simulink model "MICROBOT_1_backup"  (R2015a)
settings: Solver=ode45  StartTime=0.0  StopTime=inf  FixedStep=0.001  RelTol=1e-3
values from neighbouring files (symbols this model uses):
  s = serial('COM4','BaudRate',9600,'DataBits', 8,'Terminator',13)    [start.m]
undefined symbols (not defined in the file or in its folder): board, MICROBOT_1, RootGround, RootPart, W01_2, W02_1, W03_1, W04, W05, W06, W07, W08
libraries: mblibv1 x39
settings Model: Creator=anhkh  LastModifiedBy=anhkh
settings SimMechanicsCC: VisOnUpdateDiagram=on  VisDuringSimulation=on

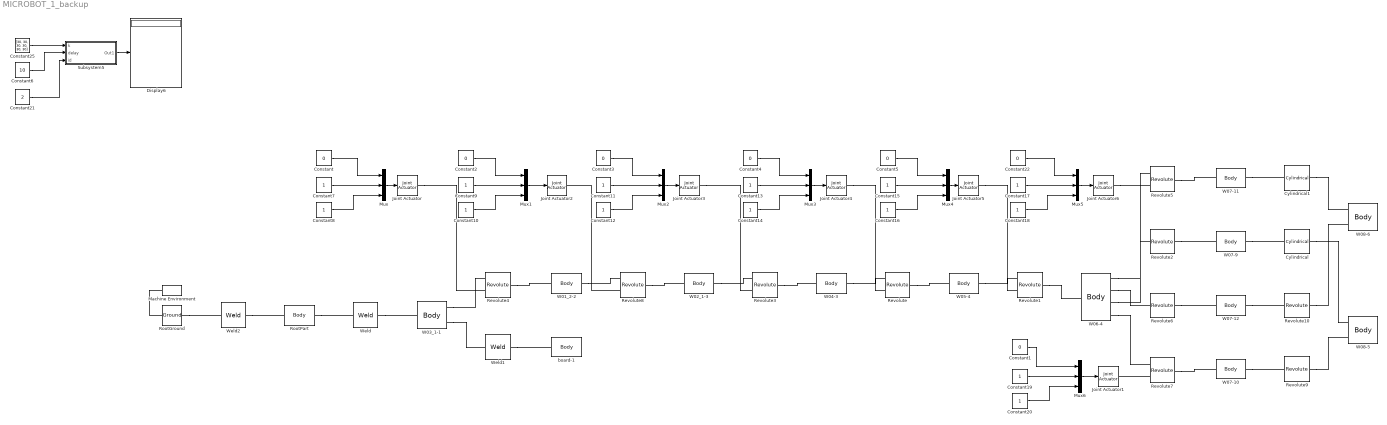
== system MICROBOT_1_backup ==
  Constant{,1..5,22} (7 alike) : Constant  Value=0
  Constant{7..20} (14 alike) : Constant
  Constant21 : Constant  Value=2
  Constant25 : Constant  Value=[30, 30, 30, 30, 30, 30]
  Constant6 : Constant  Value=10
  Cylindrical : mblibv1/Joints/Cylindrical  LConnTagsString=__newl0  RConnTagsString=__newr0  UpdateFromCAD=on  PMImportedID=W07-9:-:W08-5  NumSAPorts=0  CutJoint=off  MarkAsCut=off  Primitives=prismatic  PrimitiveProps=P1$WORLD$[0.0885398,3.2164e-12,0.996073]$prismatic#R1$WORLD$[0.0885398,3.21611e-12,0.996073]$revolute  DialogClass=JointBlock  P1Axis=[0.0885398,3.2164e-12,0.996073]  R1Axis=[0.0885398,3.21611e-12,0.996073]
  Cylindrical1 : mblibv1/Joints/Cylindrical  LConnTagsString=__newl0  RConnTagsString=__newr0  UpdateFromCAD=on  PMImportedID=W07-11:-:W08-6  NumSAPorts=0  CutJoint=off  MarkAsCut=off  Primitives=prismatic  PrimitiveProps=P1$WORLD$[-0.0885398,-3.21743e-12,-0.996073]$prismatic#R1$WORLD$[0.0885398,3.21752e-12,0.996073]$revolute  DialogClass=JointBlock  P1Axis=[-0.0885398,-3.21743e-12,-0.996073]  R1Axis=[0.0885398,3.21752e-12,0.996073]
  Display6 : Display
  Joint Actuator{,1..6} (7 alike) : mblibv1/Sensors &  Actuators/Joint Actuator  UpdateFromCAD=off  PhysicalDomain=Mechanical  PortType=blob  ActuationStyle=Motion  AngleUnits=deg  ArcVelocityUnits=deg/s  ArcAccelerationUnits=deg/s^2  CoordPositionUnits=m  VelocityUnits=m/s  AccelerationUnits=m/s^2  ForceUnits=N  TorqueUnits=N*m  ActiveIO=on  Width=3  DialogClass=MechanicalActuatorBlock  Primitive=R1  ReferenceFrame=Absolute (World)
  Machine Environment : mblibv1/Bodies/Machine Environment  PortType=env  PhysicalDomain=Mechanical  DialogTemplateClass=MECH.MachineEnvironment  SyncWhenCopied=off  Gravity=[0 -9.81 0]  GravityUnits=m/s^2  GravityAsSignal=off  Dimensionality=Auto-detect  AnalysisType=Forward dynamics  LinearAssemblyTolerance=1e-3  LinearAssemblyToleranceUnits=m  AngularAssemblyTolerance=1e-3  AngularAssemblyToleranceUnits=rad  ConstraintSolverType=Stabilizing  ConstraintRelTolerance=1e-4  ConstraintAbsTolerance=1e-4  UseRobustSingularityHandling=off  RedundancyAnalysisToleranceType=Automatically select tolerance  RedundancyAnalysisTolerance=1e-14  StatePerturbationType=Fixed  PerturbationSize=1e-5  VisualizeMachine=on  BodyVisualizationType=Use model default body geometries  BodyColorSelMode=Use model default  DefaultBodyColor=[1 0 0]
  Mux{,1..6} (7 alike) : Mux  Inputs=3
  Revolute : mblibv1/Joints/Revolute  LConnTagsString=__newl0|SA1  RConnTagsString=__newr0  UpdateFromCAD=on  PMImportedID=W04-3:-:W05-4  NumSAPorts=1  CutJoint=off  MarkAsCut=off  Primitives=prismatic  PrimitiveProps=R1$WORLD$[1.97265e-12,1,0]$revolute  DialogClass=JointBlock  R1Axis=[1.97265e-12,1,0]
  Revolute1 : mblibv1/Joints/Revolute  LConnTagsString=__newl0|SA1  RConnTagsString=__newr0  UpdateFromCAD=on  PMImportedID=W05-4:-:W06-4  NumSAPorts=1  CutJoint=off  MarkAsCut=off  Primitives=prismatic  PrimitiveProps=R1$WORLD$[0.996073,-1.96452e-12,-0.0885398]$revolute  DialogClass=JointBlock  R1Axis=[0.996073,-1.96452e-12,-0.0885398]
  Revolute10 : mblibv1/Joints/Revolute  LConnTagsString=__newl0  RConnTagsString=__newr0  UpdateFromCAD=on  PMImportedID=W07-12:-:W08-6  NumSAPorts=0  CutJoint=off  MarkAsCut=off  Primitives=prismatic  PrimitiveProps=R1$WORLD$[0.0885398,3.21754e-12,0.996073]$revolute  DialogClass=JointBlock  R1Axis=[0.0885398,3.21754e-12,0.996073]
  Revolute2 : mblibv1/Joints/Revolute  LConnTagsString=__newl0  RConnTagsString=__newr0  UpdateFromCAD=on  PMImportedID=W06-4:-:W07-9  NumSAPorts=0  CutJoint=off  MarkAsCut=off  Primitives=prismatic  PrimitiveProps=R1$WORLD$[-0.0885398,-3.21743e-12,-0.996073]$revolute  DialogClass=JointBlock  R1Axis=[-0.0885398,-3.21743e-12,-0.996073]
  Revolute3 : mblibv1/Joints/Revolute  LConnTagsString=__newl0|SA1  RConnTagsString=__newr0  UpdateFromCAD=on  PMImportedID=W02_1-3:-:W04-3  NumSAPorts=1  CutJoint=off  MarkAsCut=off  Primitives=prismatic  PrimitiveProps=R1$WORLD$[1.97263e-12,1,0]$revolute  DialogClass=JointBlock  R1Axis=[1.97263e-12,1,0]
  Revolute4 : mblibv1/Joints/Revolute  LConnTagsString=__newl0|SA1  RConnTagsString=__newr0  UpdateFromCAD=on  PMImportedID=W01_2-2:-:W03_1-1  NumSAPorts=1  CutJoint=off  MarkAsCut=off  Primitives=prismatic  PrimitiveProps=R1$WORLD$[0,0,-1]$revolute  DialogClass=JointBlock  R1Axis=[0,0,-1]
  Revolute5 : mblibv1/Joints/Revolute  LConnTagsString=__newl0|SA1  RConnTagsString=__newr0  UpdateFromCAD=on  PMImportedID=W06-4:-:W07-11  NumSAPorts=1  CutJoint=off  MarkAsCut=off  Primitives=prismatic  PrimitiveProps=R1$WORLD$[-0.0885398,-3.21743e-12,-0.996073]$revolute  DialogClass=JointBlock  R1Axis=[-0.0885398,-3.21743e-12,-0.996073]
  Revolute6 : mblibv1/Joints/Revolute  LConnTagsString=__newl0  RConnTagsString=__newr0  UpdateFromCAD=on  PMImportedID=W06-4:-:W07-12  NumSAPorts=0  CutJoint=off  MarkAsCut=off  Primitives=prismatic  PrimitiveProps=R1$WORLD$[-0.0885398,-3.21743e-12,-0.996073]$revolute  DialogClass=JointBlock  R1Axis=[-0.0885398,-3.21743e-12,-0.996073]
  Revolute7 : mblibv1/Joints/Revolute  LConnTagsString=__newl0|SA1  RConnTagsString=__newr0  UpdateFromCAD=on  PMImportedID=W06-4:-:W07-10  NumSAPorts=1  CutJoint=off  MarkAsCut=off  Primitives=prismatic  PrimitiveProps=R1$WORLD$[-0.0885398,-3.21743e-12,-0.996073]$revolute  DialogClass=JointBlock  R1Axis=[-0.0885398,-3.21743e-12,-0.996073]
  Revolute8 : mblibv1/Joints/Revolute  LConnTagsString=__newl0|SA1  RConnTagsString=__newr0  UpdateFromCAD=on  PMImportedID=W01_2-2:-:W02_1-3  NumSAPorts=1  CutJoint=off  MarkAsCut=off  Primitives=prismatic  PrimitiveProps=R1$WORLD$[-1.9721e-12,-1,0]$revolute  DialogClass=JointBlock  R1Axis=[-1.9721e-12,-1,0]
  Revolute9 : mblibv1/Joints/Revolute  LConnTagsString=__newl0  RConnTagsString=__newr0  UpdateFromCAD=on  PMImportedID=W07-10:-:W08-5  NumSAPorts=0  CutJoint=off  MarkAsCut=off  Primitives=prismatic  PrimitiveProps=R1$WORLD$[0.0885398,3.2164e-12,0.996073]$revolute  DialogClass=JointBlock  R1Axis=[0.0885398,3.2164e-12,0.996073]
  RootGround : mblibv1/Bodies/Ground  UpdateFromCAD=on  PMImportedID=RootGround  LeftPortType=env  RightPortType=workingframe  PhysicalDomain=Mechanical  DialogClass=GroundBlock  CoordPosition=[-0.110803,0.40847,0.0544949]  CoordPositionUnits=m  StateVectorMgrId=3  MachineId=[4 0]  ShowEnvPort=on  ParameterChecksum=[2064798137, 1484770623, 251117345, 3844192694]  TopologyChecksum=[3823588316, 2441359055, 4135265906, 3916664184]
  RootPart : mblibv1/Bodies/Body  LConnTagsString=CS3  RConnTagsString=CS2  UpdateFromCAD=on  PMImportedID=MICROBOT_1/RootPart  DialogClass=MechanicalBodyBlock  Mass=0  MassUnits=kg  InertiaUnits=kg*m^2  Inertia=[0,0,0;0,0,0;0,0,0]  Shape=Cylinder  ShapeDims=[1 1]  ShapeUnits=m  ShapeUse=false  Density=1  DensityUnits=kg/m^3  DensityUse=false  GraphicsMode=MACHINE_DEFAULT  BodyColorSelMode=MACHINE_DEFAULT  BodyColor=[1;0;0]  AttachedToCS=CS1  CG=Right$CG$[-0.110803 0.40847 0.0544949]$WORLD$WORLD$m$[1 0 0;0 1 0;0 0 1]$3x3 Transform$rad$WORLD$false$MICROBOT_1/RootPart::CG(AUTOGEN)  WorkingFrames=Right$CS1$[0 0 0]$WORLD$WORLD$m$[1 0 0;0 1 0;0 0 1]$3x3 Transform$rad$WORLD$false$MICROBOT_1/RootPart::CS1(AUTOGEN)#Right$CS2$[-0.107087 0.143871 0.0371879]$WORLD$WORLD$m$[1 0 0;0 1 0;0 0 1]$3x3 Transform$rad$WORLD$true$MICROBOT_1/RootPart:-:W03_1-1::MICROBOT_1/RootPart(AUTOGEN)#Left$CS3$[-0.110803 0.40847 0.0544949]$WORLD$WORLD$m$[1 0 0;0 1 0;0 0 1]$3x3 Transform$rad$WORLD$true$MICROBOT_1/RootPart:-:RootGround::MICROBOT_1/RootPart(AUTOGEN)  CGPos=[-0.110803 0.40847 0.0544949]  CGRot=[1 0 0;0 1 0;0 0 1]  CS0Pos=[]  CS0Rot=[]  CS1Pos=[0 0 0]  CS1Rot=[1 0 0;0 1 0;0 0 1]  CS2Pos=[-0.107087 0.143871 0.0371879]  CS2Rot=[1 0 0;0 1 0;0 0 1]  CS3Pos=[-0.110803 0.40847 0.0544949]  CS3Rot=[1 0 0;0 1 0;0 0 1]  CS4Pos=[]  CS4Rot=[]  CS5Pos=[]  CS5Rot=[]  CS6Pos=[]  CS6Rot=[]  CS7Pos=[]  CS7Rot=[]  CS8Pos=[]  CS8Rot=[]  CS9Pos=[]  CS9Rot=[]  CS10Pos=[]  CS10Rot=[]  CS11Pos=[]  CS11Rot=[]  CS12Pos=[]  CS12Rot=[]  CS13Pos=[]  CS13Rot=[]  CS14Pos=[]  CS14Rot=[]  CS15Pos=[]  CS15Rot=[]  CS16Pos=[]  CS16Rot=[]  CS17Pos=[]  CS17Rot=[]  CS18Pos=[]  CS18Rot=[]  CS19Pos=[]  CS19Rot=[]  CS20Pos=[]  CS20Rot=[]
  Subsystem5 : Subsystem
  W01_2-2 : mblibv1/Bodies/Body  LConnTagsString=CS3  RConnTagsString=CS2  UpdateFromCAD=on  PMImportedID=W01_2-2  DialogClass=MechanicalBodyBlock  Mass=3.41752  MassUnits=kg  InertiaUnits=kg*m^2  Inertia=[0.0156091,-9.74217e-10,-8.96339e-09;-9.74217e-10,0.0136555,0.00112438;-8.96339e-09,0.00112438,0.0159365]  Shape=Cylinder  ShapeDims=[1 1]  ShapeUnits=m  ShapeUse=false  Density=1  DensityUnits=kg/m^3  DensityUse=false  GraphicsMode=GFXFILE  GraphicsFileName=MICROBOT_1 - W01_2-2.STL  BodyColorSelMode=COLORPALETTE  BodyColor=[0.792157;0.819608;0.933333]  AttachedToCS=CS1  CG=Right$CG$[-0.15354 0.221184 0.150881]$WORLD$WORLD$m$[1.9721e-12 1 0;1 -1.9721e-12 0;0 0 -1]$3x3 Transform$rad$WORLD$false$W01_2-2::CG(AUTOGEN)  WorkingFrames=Right$CS1$[-0.157087 0.221184 0.193]$WORLD$WORLD$m$[1.9721e-12 1 0;1 -1.9721e-12 0;0 0 -1]$3x3 Transform$rad$WORLD$false$W01_2-2::CS1(AUTOGEN)#Right$CS2$[-0.107087 0.252684 0.243]$WORLD$WORLD$m$[1 0 0;0 1 0;0 0 1]$3x3 Transform$rad$WORLD$true$W01_2-2:-:W02_1-3::W01_2-2(AUTOGEN)#Left$CS3$[-0.107087 0.221184 0.103]$WORLD$WORLD$m$[1 0 0;0 1 0;0 0 1]$3x3 Transform$rad$WORLD$true$W01_2-2:-:W03_1-1::W01_2-2(AUTOGEN)  CGPos=[-0.15354 0.221184 0.150881]  CGRot=[1.9721e-12 1 0;1 -1.9721e-12 0;0 0 -1]  CS0Pos=[]  CS0Rot=[]  CS1Pos=[-0.157087 0.221184 0.193]  CS1Rot=[1.9721e-12 1 0;1 -1.9721e-12 0;0 0 -1]  CS2Pos=[-0.107087 0.252684 0.243]  CS2Rot=[1 0 0;0 1 0;0 0 1]  CS3Pos=[-0.107087 0.221184 0.103]  CS3Rot=[1 0 0;0 1 0;0 0 1]  CS4Pos=[]  CS4Rot=[]  CS5Pos=[]  CS5Rot=[]  CS6Pos=[]  CS6Rot=[]  CS7Pos=[]  CS7Rot=[]  CS8Pos=[]  CS8Rot=[]  CS9Pos=[]  CS9Rot=[]  CS10Pos=[]  CS10Rot=[]  CS11Pos=[]  CS11Rot=[]  CS12Pos=[]  CS12Rot=[]  CS13Pos=[]  CS13Rot=[]  CS14Pos=[]  CS14Rot=[]  CS15Pos=[]  CS15Rot=[]  CS16Pos=[]  CS16Rot=[]  CS17Pos=[]  CS17Rot=[]  CS18Pos=[]  CS18Rot=[]  CS19Pos=[]  CS19Rot=[]  CS20Pos=[]  CS20Rot=[]
  W02_1-3 : mblibv1/Bodies/Body  LConnTagsString=CS2  RConnTagsString=CS3  UpdateFromCAD=on  PMImportedID=W02_1-3  DialogClass=MechanicalBodyBlock  Mass=0.137184  MassUnits=kg  InertiaUnits=kg*m^2  Inertia=[0.000250835,-0.000173843,-1.3272e-07;-0.000173843,0.000692155,9.67815e-08;-1.3272e-07,9.67815e-08,0.000724516]  Shape=Cylinder  ShapeDims=[1 1]  ShapeUnits=m  ShapeUse=false  Density=1  DensityUnits=kg/m^3  DensityUse=false  GraphicsMode=GFXFILE  GraphicsFileName=MICROBOT_1 - W02_1-3.STL  BodyColorSelMode=COLORPALETTE  BodyColor=[0.792157;0.819608;0.933333]  AttachedToCS=CS1  CG=Right$CG$[-0.0248881 0.22102 0.249502]$WORLD$WORLD$m$[0.948668 0.316273 -1.97263e-12;-1.86984e-12 0 -1;-0.316273 0.948668 0]$3x3 Transform$rad$WORLD$false$W02_1-3::CG(AUTOGEN)  WorkingFrames=Right$CS1$[-0.0240745 0.252684 0.238257]$WORLD$WORLD$m$[0.948668 0.316273 -1.97263e-12;-1.86984e-12 0 -1;-0.316273 0.948668 0]$3x3 Transform$rad$WORLD$false$W02_1-3::CS1(AUTOGEN)#Left$CS2$[-0.107087 0.252684 0.243]$WORLD$WORLD$m$[1 0 0;0 1 0;0 0 1]$3x3 Transform$rad$WORLD$true$W01_2-2:-:W02_1-3::W02_1-3(AUTOGEN)#Right$CS3$[0.0779125 0.236184 0.243]$WORLD$WORLD$m$[1 0 0;0 1 0;0 0 1]$3x3 Transform$rad$WORLD$true$W02_1-3:-:W04-3::W02_1-3(AUTOGEN)  CGPos=[-0.0248881 0.22102 0.249502]  CGRot=[0.948668 0.316273 -1.97263e-12;-1.86984e-12 0 -1;-0.316273 0.948668 0]  CS0Pos=[]  CS0Rot=[]  CS1Pos=[-0.0240745 0.252684 0.238257]  CS1Rot=[0.948668 0.316273 -1.97263e-12;-1.86984e-12 0 -1;-0.316273 0.948668 0]  CS2Pos=[-0.107087 0.252684 0.243]  CS2Rot=[1 0 0;0 1 0;0 0 1]  CS3Pos=[0.0779125 0.236184 0.243]  CS3Rot=[1 0 0;0 1 0;0 0 1]  CS4Pos=[]  CS4Rot=[]  CS5Pos=[]  CS5Rot=[]  CS6Pos=[]  CS6Rot=[]  CS7Pos=[]  CS7Rot=[]  CS8Pos=[]  CS8Rot=[]  CS9Pos=[]  CS9Rot=[]  CS10Pos=[]  CS10Rot=[]  CS11Pos=[]  CS11Rot=[]  CS12Pos=[]  CS12Rot=[]  CS13Pos=[]  CS13Rot=[]  CS14Pos=[]  CS14Rot=[]  CS15Pos=[]  CS15Rot=[]  CS16Pos=[]  CS16Rot=[]  CS17Pos=[]  CS17Rot=[]  CS18Pos=[]  CS18Rot=[]  CS19Pos=[]  CS19Rot=[]  CS20Pos=[]  CS20Rot=[]
  W03_1-1 : mblibv1/Bodies/Body  LConnTagsString=CS2  RConnTagsString=CS3|CS4  UpdateFromCAD=on  PMImportedID=W03_1-1  DialogClass=MechanicalBodyBlock  Mass=3.89994  MassUnits=kg  InertiaUnits=kg*m^2  Inertia=[0.0172249,0,0;0,0.0322437,-3.95609e-05;0,-3.95609e-05,0.0192496]  Shape=Cylinder  ShapeDims=[1 1]  ShapeUnits=m  ShapeUse=false  Density=1  DensityUnits=kg/m^3  DensityUse=false  GraphicsMode=GFXFILE  GraphicsFileName=MICROBOT_1 - W03_1-1.STL  BodyColorSelMode=COLORPALETTE  BodyColor=[0.792157;0.819608;0.933333]  AttachedToCS=CS1  CG=Right$CG$[-0.107087 0.143871 0.0371879]$WORLD$WORLD$m$[-1 0 0;0 0 1;0 1 0]$3x3 Transform$rad$WORLD$false$W03_1-1::CG(AUTOGEN)  WorkingFrames=Right$CS1$[-0.107087 0.036184 0.04]$WORLD$WORLD$m$[-1 0 0;0 0 1;0 1 0]$3x3 Transform$rad$WORLD$false$W03_1-1::CS1(AUTOGEN)#Left$CS2$[-0.107087 0.143871 0.0371879]$WORLD$WORLD$m$[1 0 0;0 1 0;0 0 1]$3x3 Transform$rad$WORLD$true$MICROBOT_1/RootPart:-:W03_1-1::W03_1-1(AUTOGEN)#Right$CS3$[-0.107087 0.221184 0.103]$WORLD$WORLD$m$[1 0 0;0 1 0;0 0 1]$3x3 Transform$rad$WORLD$true$W01_2-2:-:W03_1-1::W03_1-1(AUTOGEN)#Right$CS4$[-0.107087 0.036184 -0.02]$WORLD$WORLD$m$[1 0 0;0 1 0;0 0 1]$3x3 Transform$rad$WORLD$true$W03_1-1:-:board-1::W03_1-1(AUTOGEN)  CGPos=[-0.107087 0.143871 0.0371879]  CGRot=[-1 0 0;0 0 1;0 1 0]  CS0Pos=[]  CS0Rot=[]  CS1Pos=[-0.107087 0.036184 0.04]  CS1Rot=[-1 0 0;0 0 1;0 1 0]  CS2Pos=[-0.107087 0.143871 0.0371879]  CS2Rot=[1 0 0;0 1 0;0 0 1]  CS3Pos=[-0.107087 0.221184 0.103]  CS3Rot=[1 0 0;0 1 0;0 0 1]  CS4Pos=[-0.107087 0.036184 -0.02]  CS4Rot=[1 0 0;0 1 0;0 0 1]  CS5Pos=[]  CS5Rot=[]  CS6Pos=[]  CS6Rot=[]  CS7Pos=[]  CS7Rot=[]  CS8Pos=[]  CS8Rot=[]  CS9Pos=[]  CS9Rot=[]  CS10Pos=[]  CS10Rot=[]  CS11Pos=[]  CS11Rot=[]  CS12Pos=[]  CS12Rot=[]  CS13Pos=[]  CS13Rot=[]  CS14Pos=[]  CS14Rot=[]  CS15Pos=[]  CS15Rot=[]  CS16Pos=[]  CS16Rot=[]  CS17Pos=[]  CS17Rot=[]  CS18Pos=[]  CS18Rot=[]  CS19Pos=[]  CS19Rot=[]  CS20Pos=[]  CS20Rot=[]
  W04-3 : mblibv1/Bodies/Body  LConnTagsString=CS2  RConnTagsString=CS3  UpdateFromCAD=on  PMImportedID=W04-3  DialogClass=MechanicalBodyBlock  Mass=0.028469  MassUnits=kg  InertiaUnits=kg*m^2  Inertia=[0.00010055,-1.1564e-07,2.98034e-07;-1.1564e-07,0.000108696,-6.97188e-07;2.98034e-07,-6.97188e-07,2.10954e-05]  Shape=Cylinder  ShapeDims=[1 1]  ShapeUnits=m  ShapeUse=false  Density=1  DensityUnits=kg/m^3  DensityUse=false  GraphicsMode=GFXFILE  GraphicsFileName=MICROBOT_1 - W04-3.STL  BodyColorSelMode=COLORPALETTE  BodyColor=[0.792157;0.819608;0.933333]  AttachedToCS=CS1  CG=Right$CG$[0.00168848 0.221868 0.236562]$WORLD$WORLD$m$[1.97265e-12 0 1;1 0 -1.97265e-12;0 1 0]$3x3 Transform$rad$WORLD$false$W04-3::CG(AUTOGEN)  WorkingFrames=Right$CS1$[0.0779125 0.221184 0.243]$WORLD$WORLD$m$[1.97265e-12 0 1;1 0 -1.97265e-12;0 1 0]$3x3 Transform$rad$WORLD$false$W04-3::CS1(AUTOGEN)#Left$CS2$[0.0779125 0.236184 0.243]$WORLD$WORLD$m$[1 0 0;0 1 0;0 0 1]$3x3 Transform$rad$WORLD$true$W02_1-3:-:W04-3::W04-3(AUTOGEN)#Right$CS3$[-0.102087 0.247184 0.243]$WORLD$WORLD$m$[1 0 0;0 1 0;0 0 1]$3x3 Transform$rad$WORLD$true$W04-3:-:W05-4::W04-3(AUTOGEN)  CGPos=[0.00168848 0.221868 0.236562]  CGRot=[1.97265e-12 0 1;1 0 -1.97265e-12;0 1 0]  CS0Pos=[]  CS0Rot=[]  CS1Pos=[0.0779125 0.221184 0.243]  CS1Rot=[1.97265e-12 0 1;1 0 -1.97265e-12;0 1 0]  CS2Pos=[0.0779125 0.236184 0.243]  CS2Rot=[1 0 0;0 1 0;0 0 1]  CS3Pos=[-0.102087 0.247184 0.243]  CS3Rot=[1 0 0;0 1 0;0 0 1]  CS4Pos=[]  CS4Rot=[]  CS5Pos=[]  CS5Rot=[]  CS6Pos=[]  CS6Rot=[]  CS7Pos=[]  CS7Rot=[]  CS8Pos=[]  CS8Rot=[]  CS9Pos=[]  CS9Rot=[]  CS10Pos=[]  CS10Rot=[]  CS11Pos=[]  CS11Rot=[]  CS12Pos=[]  CS12Rot=[]  CS13Pos=[]  CS13Rot=[]  CS14Pos=[]  CS14Rot=[]  CS15Pos=[]  CS15Rot=[]  CS16Pos=[]  CS16Rot=[]  CS17Pos=[]  CS17Rot=[]  CS18Pos=[]  CS18Rot=[]  CS19Pos=[]  CS19Rot=[]  CS20Pos=[]  CS20Rot=[]
  W05-4 : mblibv1/Bodies/Body  LConnTagsString=CS2  RConnTagsString=CS3  UpdateFromCAD=on  PMImportedID=W05-4  DialogClass=MechanicalBodyBlock  Mass=0.0114047  MassUnits=kg  InertiaUnits=kg*m^2  Inertia=[7.08852e-07,0,6.72492e-12;0,1.28223e-06,-2.77128e-11;6.72492e-12,-2.77128e-11,1.23052e-06]  Shape=Cylinder  ShapeDims=[1 1]  ShapeUnits=m  ShapeUse=false  Density=1  DensityUnits=kg/m^3  DensityUse=false  GraphicsMode=GFXFILE  GraphicsFileName=MICROBOT_1 - W05-4.STL  BodyColorSelMode=COLORPALETTE  BodyColor=[0.792157;0.819608;0.933333]  AttachedToCS=CS1  CG=Right$CG$[-0.102528 0.221184 0.243039]$WORLD$WORLD$m$[1.97271e-12 -0.996073 0.0885398;1 1.96452e-12 0;0 0.0885398 0.996073]$3x3 Transform$rad$WORLD$false$W05-4::CG(AUTOGEN)  WorkingFrames=Right$CS1$[-0.102087 0.221184 0.243]$WORLD$WORLD$m$[1.97271e-12 -0.996073 0.0885398;1 1.96452e-12 0;0 0.0885398 0.996073]$3x3 Transform$rad$WORLD$false$W05-4::CS1(AUTOGEN)#Left$CS2$[-0.102087 0.247184 0.243]$WORLD$WORLD$m$[1 0 0;0 1 0;0 0 1]$3x3 Transform$rad$WORLD$true$W04-3:-:W05-4::W05-4(AUTOGEN)#Right$CS3$[-0.103979 0.221184 0.243168]$WORLD$WORLD$m$[1 0 0;0 1 0;0 0 1]$3x3 Transform$rad$WORLD$true$W05-4:-:W06-4::W05-4(AUTOGEN)  CGPos=[-0.102528 0.221184 0.243039]  CGRot=[1.97271e-12 -0.996073 0.0885398;1 1.96452e-12 0;0 0.0885398 0.996073]  CS0Pos=[]  CS0Rot=[]  CS1Pos=[-0.102087 0.221184 0.243]  CS1Rot=[1.97271e-12 -0.996073 0.0885398;1 1.96452e-12 0;0 0.0885398 0.996073]  CS2Pos=[-0.102087 0.247184 0.243]  CS2Rot=[1 0 0;0 1 0;0 0 1]  CS3Pos=[-0.103979 0.221184 0.243168]  CS3Rot=[1 0 0;0 1 0;0 0 1]  CS4Pos=[]  CS4Rot=[]  CS5Pos=[]  CS5Rot=[]  CS6Pos=[]  CS6Rot=[]  CS7Pos=[]  CS7Rot=[]  CS8Pos=[]  CS8Rot=[]  CS9Pos=[]  CS9Rot=[]  CS10Pos=[]  CS10Rot=[]  CS11Pos=[]  CS11Rot=[]  CS12Pos=[]  CS12Rot=[]  CS13Pos=[]  CS13Rot=[]  CS14Pos=[]  CS14Rot=[]  CS15Pos=[]  CS15Rot=[]  CS16Pos=[]  CS16Rot=[]  CS17Pos=[]  CS17Rot=[]  CS18Pos=[]  CS18Rot=[]  CS19Pos=[]  CS19Rot=[]  CS20Pos=[]  CS20Rot=[]
  W06-4 : mblibv1/Bodies/Body  LConnTagsString=CS3  RConnTagsString=CS2|CS4|CS5|CS6  UpdateFromCAD=on  PMImportedID=W06-4  DialogClass=MechanicalBodyBlock  Mass=0.00360366  MassUnits=kg  InertiaUnits=kg*m^2  Inertia=[3.16611e-07,4.38162e-09,0;4.38162e-09,1.36274e-06,0;0,0,1.31379e-06]  Shape=Cylinder  ShapeDims=[1 1]  ShapeUnits=m  ShapeUse=false  Density=1  DensityUnits=kg/m^3  DensityUse=false  GraphicsMode=GFXFILE  GraphicsFileName=MICROBOT_1 - W06-4.STL  BodyColorSelMode=COLORPALETTE  BodyColor=[0.792157;0.819608;0.933333]  AttachedToCS=CS1  CG=Right$CG$[-0.0815589 0.221054 0.241175]$WORLD$WORLD$m$[-1.34635e-12 -0.996073 -0.0885398;-1 1.63765e-12 -3.21743e-12;3.34979e-12 0.0885398 -0.996073]$3x3 Transform$rad$WORLD$false$W06-4::CG(AUTOGEN)  WorkingFrames=Right$CS1$[-0.0770144 0.221184 0.240771]$WORLD$WORLD$m$[-1.34635e-12 -0.996073 -0.0885398;-1 1.63765e-12 -3.21743e-12;3.34979e-12 0.0885398 -0.996073]$3x3 Transform$rad$WORLD$false$W06-4::CS1(AUTOGEN)#Right$CS2$[-0.0797149 0.199184 0.23298]$WORLD$WORLD$m$[1 0 0;0 1 0;0 0 1]$3x3 Transform$rad$WORLD$true$W06-4:-:W07-11::W06-4(AUTOGEN)#Left$CS3$[-0.103979 0.221184 0.243168]$WORLD$WORLD$m$[1 0 0;0 1 0;0 0 1]$3x3 Transform$rad$WORLD$true$W05-4:-:W06-4::W06-4(AUTOGEN)#Right$CS4$[-0.0797149 0.191184 0.23298]$WORLD$WORLD$m$[1 0 0;0 1 0;0 0 1]$3x3 Transform$rad$WORLD$true$W06-4:-:W07-12::W06-4(AUTOGEN)#Right$CS5$[-0.0797149 0.251184 0.23298]$WORLD$WORLD$m$[1 0 0;0 1 0;0 0 1]$3x3 Transform$rad$WORLD$true$W06-4:-:W07-9::W06-4(AUTOGEN)#Right$CS6$[-0.0797149 0.243184 0.23298]$WORLD$WORLD$m$[1 0 0;0 1 0;0 0 1]$3x3 Transform$rad$WORLD$true$W06-4:-:W07-10::W06-4(AUTOGEN)  CGPos=[-0.0815589 0.221054 0.241175]  CGRot=[-1.34635e-12 -0.996073 -0.0885398;-1 1.63765e-12 -3.21743e-12;3.34979e-12 0.0885398 -0.996073]  CS0Pos=[]  CS0Rot=[]  CS1Pos=[-0.0770144 0.221184 0.240771]  CS1Rot=[-1.34635e-12 -0.996073 -0.0885398;-1 1.63765e-12 -3.21743e-12;3.34979e-12 0.0885398 -0.996073]  CS2Pos=[-0.0797149 0.199184 0.23298]  CS2Rot=[1 0 0;0 1 0;0 0 1]  CS3Pos=[-0.103979 0.221184 0.243168]  CS3Rot=[1 0 0;0 1 0;0 0 1]  CS4Pos=[-0.0797149 0.191184 0.23298]  CS4Rot=[1 0 0;0 1 0;0 0 1]  CS5Pos=[-0.0797149 0.251184 0.23298]  CS5Rot=[1 0 0;0 1 0;0 0 1]  CS6Pos=[-0.0797149 0.243184 0.23298]  CS6Rot=[1 0 0;0 1 0;0 0 1]  CS7Pos=[]  CS7Rot=[]  CS8Pos=[]  CS8Rot=[]  CS9Pos=[]  CS9Rot=[]  CS10Pos=[]  CS10Rot=[]  CS11Pos=[]  CS11Rot=[]  CS12Pos=[]  CS12Rot=[]  CS13Pos=[]  CS13Rot=[]  CS14Pos=[]  CS14Rot=[]  CS15Pos=[]  CS15Rot=[]  CS16Pos=[]  CS16Rot=[]  CS17Pos=[]  CS17Rot=[]  CS18Pos=[]  CS18Rot=[]  CS19Pos=[]  CS19Rot=[]  CS20Pos=[]  CS20Rot=[]
  W07-10 : mblibv1/Bodies/Body  LConnTagsString=CS2  RConnTagsString=CS3  UpdateFromCAD=on  PMImportedID=W07-10  DialogClass=MechanicalBodyBlock  Mass=0.00554345  MassUnits=kg  InertiaUnits=kg*m^2  Inertia=[1.25755e-06,0,0;0,1.41119e-07,0;0,0,1.16215e-06]  Shape=Cylinder  ShapeDims=[1 1]  ShapeUnits=m  ShapeUse=false  Density=1  DensityUnits=kg/m^3  DensityUse=false  GraphicsMode=GFXFILE  GraphicsFileName=MICROBOT_1 - W07-10.STL  BodyColorSelMode=COLORPALETTE  BodyColor=[0.792157;0.819608;0.933333]  AttachedToCS=CS1  CG=Right$CG$[-0.0592413 0.233684 0.239191]$WORLD$WORLD$m$[-0.430122 -0.898418 -0.0885398;-0.901961 0.431818 -3.2164e-12;0.0382331 0.0798594 -0.996073]$3x3 Transform$rad$WORLD$false$W07-10::CG(AUTOGEN)  WorkingFrames=Right$CS1$[-0.0587101 0.233684 0.245168]$WORLD$WORLD$m$[-0.430122 -0.898418 -0.0885398;-0.901961 0.431818 -3.2164e-12;0.0382331 0.0798594 -0.996073]$3x3 Transform$rad$WORLD$false$W07-10::CS1(AUTOGEN)#Left$CS2$[-0.0797149 0.243184 0.23298]$WORLD$WORLD$m$[1 0 0;0 1 0;0 0 1]$3x3 Transform$rad$WORLD$true$W06-4:-:W07-10::W07-10(AUTOGEN)#Right$CS3$[-0.0401844 0.224184 0.229466]$WORLD$WORLD$m$[1 0 0;0 1 0;0 0 1]$3x3 Transform$rad$WORLD$true$W07-10:-:W08-5::W07-10(AUTOGEN)  CGPos=[-0.0592413 0.233684 0.239191]  CGRot=[-0.430122 -0.898418 -0.0885398;-0.901961 0.431818 -3.2164e-12;0.0382331 0.0798594 -0.996073]  CS0Pos=[]  CS0Rot=[]  CS1Pos=[-0.0587101 0.233684 0.245168]  CS1Rot=[-0.430122 -0.898418 -0.0885398;-0.901961 0.431818 -3.2164e-12;0.0382331 0.0798594 -0.996073]  CS2Pos=[-0.0797149 0.243184 0.23298]  CS2Rot=[1 0 0;0 1 0;0 0 1]  CS3Pos=[-0.0401844 0.224184 0.229466]  CS3Rot=[1 0 0;0 1 0;0 0 1]  CS4Pos=[]  CS4Rot=[]  CS5Pos=[]  CS5Rot=[]  CS6Pos=[]  CS6Rot=[]  CS7Pos=[]  CS7Rot=[]  CS8Pos=[]  CS8Rot=[]  CS9Pos=[]  CS9Rot=[]  CS10Pos=[]  CS10Rot=[]  CS11Pos=[]  CS11Rot=[]  CS12Pos=[]  CS12Rot=[]  CS13Pos=[]  CS13Rot=[]  CS14Pos=[]  CS14Rot=[]  CS15Pos=[]  CS15Rot=[]  CS16Pos=[]  CS16Rot=[]  CS17Pos=[]  CS17Rot=[]  CS18Pos=[]  CS18Rot=[]  CS19Pos=[]  CS19Rot=[]  CS20Pos=[]  CS20Rot=[]
  W07-11 : mblibv1/Bodies/Body  LConnTagsString=CS3  RConnTagsString=CS2  UpdateFromCAD=on  PMImportedID=W07-11  DialogClass=MechanicalBodyBlock  Mass=0.00554345  MassUnits=kg  InertiaUnits=kg*m^2  Inertia=[1.25755e-06,0,0;0,1.41119e-07,0;0,0,1.16215e-06]  Shape=Cylinder  ShapeDims=[1 1]  ShapeUnits=m  ShapeUse=false  Density=1  DensityUnits=kg/m^3  DensityUse=false  GraphicsMode=GFXFILE  GraphicsFileName=MICROBOT_1 - W07-11.STL  BodyColorSelMode=COLORPALETTE  BodyColor=[0.792157;0.819608;0.933333]  AttachedToCS=CS1  CG=Right$CG$[-0.0592413 0.208684 0.239191]$WORLD$WORLD$m$[0.430122 -0.898418 -0.0885398;-0.901961 -0.431818 -3.21753e-12;-0.0382331 0.0798594 -0.996073]$3x3 Transform$rad$WORLD$false$W07-11::CG(AUTOGEN)  WorkingFrames=Right$CS1$[-0.0587101 0.208684 0.245168]$WORLD$WORLD$m$[0.430122 -0.898418 -0.0885398;-0.901961 -0.431818 -3.21753e-12;-0.0382331 0.0798594 -0.996073]$3x3 Transform$rad$WORLD$false$W07-11::CS1(AUTOGEN)#Right$CS2$[-0.0401844 0.218184 0.229466]$WORLD$WORLD$m$[1 0 0;0 1 0;0 0 1]$3x3 Transform$rad$WORLD$true$W07-11:-:W08-6::W07-11(AUTOGEN)#Left$CS3$[-0.0797149 0.199184 0.23298]$WORLD$WORLD$m$[1 0 0;0 1 0;0 0 1]$3x3 Transform$rad$WORLD$true$W06-4:-:W07-11::W07-11(AUTOGEN)  CGPos=[-0.0592413 0.208684 0.239191]  CGRot=[0.430122 -0.898418 -0.0885398;-0.901961 -0.431818 -3.21753e-12;-0.0382331 0.0798594 -0.996073]  CS0Pos=[]  CS0Rot=[]  CS1Pos=[-0.0587101 0.208684 0.245168]  CS1Rot=[0.430122 -0.898418 -0.0885398;-0.901961 -0.431818 -3.21753e-12;-0.0382331 0.0798594 -0.996073]  CS2Pos=[-0.0401844 0.218184 0.229466]  CS2Rot=[1 0 0;0 1 0;0 0 1]  CS3Pos=[-0.0797149 0.199184 0.23298]  CS3Rot=[1 0 0;0 1 0;0 0 1]  CS4Pos=[]  CS4Rot=[]  CS5Pos=[]  CS5Rot=[]  CS6Pos=[]  CS6Rot=[]  CS7Pos=[]  CS7Rot=[]  CS8Pos=[]  CS8Rot=[]  CS9Pos=[]  CS9Rot=[]  CS10Pos=[]  CS10Rot=[]  CS11Pos=[]  CS11Rot=[]  CS12Pos=[]  CS12Rot=[]  CS13Pos=[]  CS13Rot=[]  CS14Pos=[]  CS14Rot=[]  CS15Pos=[]  CS15Rot=[]  CS16Pos=[]  CS16Rot=[]  CS17Pos=[]  CS17Rot=[]  CS18Pos=[]  CS18Rot=[]  CS19Pos=[]  CS19Rot=[]  CS20Pos=[]  CS20Rot=[]
  W07-12 : mblibv1/Bodies/Body  LConnTagsString=CS3  RConnTagsString=CS2  UpdateFromCAD=on  PMImportedID=W07-12  DialogClass=MechanicalBodyBlock  Mass=0.00554345  MassUnits=kg  InertiaUnits=kg*m^2  Inertia=[1.25755e-06,0,0;0,1.41119e-07,0;0,0,1.16215e-06]  Shape=Cylinder  ShapeDims=[1 1]  ShapeUnits=m  ShapeUse=false  Density=1  DensityUnits=kg/m^3  DensityUse=false  GraphicsMode=GFXFILE  GraphicsFileName=MICROBOT_1 - W07-12.STL  BodyColorSelMode=COLORPALETTE  BodyColor=[0.792157;0.819608;0.933333]  AttachedToCS=CS1  CG=Right$CG$[-0.0592413 0.200684 0.239191]$WORLD$WORLD$m$[0.430122 -0.898418 -0.0885398;-0.901961 -0.431818 -3.21755e-12;-0.0382331 0.0798594 -0.996073]$3x3 Transform$rad$WORLD$false$W07-12::CG(AUTOGEN)  WorkingFrames=Right$CS1$[-0.0587101 0.200684 0.245168]$WORLD$WORLD$m$[0.430122 -0.898418 -0.0885398;-0.901961 -0.431818 -3.21755e-12;-0.0382331 0.0798594 -0.996073]$3x3 Transform$rad$WORLD$false$W07-12::CS1(AUTOGEN)#Right$CS2$[-0.0401844 0.210184 0.229466]$WORLD$WORLD$m$[1 0 0;0 1 0;0 0 1]$3x3 Transform$rad$WORLD$true$W07-12:-:W08-6::W07-12(AUTOGEN)#Left$CS3$[-0.0797149 0.191184 0.23298]$WORLD$WORLD$m$[1 0 0;0 1 0;0 0 1]$3x3 Transform$rad$WORLD$true$W06-4:-:W07-12::W07-12(AUTOGEN)  CGPos=[-0.0592413 0.200684 0.239191]  CGRot=[0.430122 -0.898418 -0.0885398;-0.901961 -0.431818 -3.21755e-12;-0.0382331 0.0798594 -0.996073]  CS0Pos=[]  CS0Rot=[]  CS1Pos=[-0.0587101 0.200684 0.245168]  CS1Rot=[0.430122 -0.898418 -0.0885398;-0.901961 -0.431818 -3.21755e-12;-0.0382331 0.0798594 -0.996073]  CS2Pos=[-0.0401844 0.210184 0.229466]  CS2Rot=[1 0 0;0 1 0;0 0 1]  CS3Pos=[-0.0797149 0.191184 0.23298]  CS3Rot=[1 0 0;0 1 0;0 0 1]  CS4Pos=[]  CS4Rot=[]  CS5Pos=[]  CS5Rot=[]  CS6Pos=[]  CS6Rot=[]  CS7Pos=[]  CS7Rot=[]  CS8Pos=[]  CS8Rot=[]  CS9Pos=[]  CS9Rot=[]  CS10Pos=[]  CS10Rot=[]  CS11Pos=[]  CS11Rot=[]  CS12Pos=[]  CS12Rot=[]  CS13Pos=[]  CS13Rot=[]  CS14Pos=[]  CS14Rot=[]  CS15Pos=[]  CS15Rot=[]  CS16Pos=[]  CS16Rot=[]  CS17Pos=[]  CS17Rot=[]  CS18Pos=[]  CS18Rot=[]  CS19Pos=[]  CS19Rot=[]  CS20Pos=[]  CS20Rot=[]
  W07-9 : mblibv1/Bodies/Body  LConnTagsString=CS2  RConnTagsString=CS3  UpdateFromCAD=on  PMImportedID=W07-9  DialogClass=MechanicalBodyBlock  Mass=0.00554345  MassUnits=kg  InertiaUnits=kg*m^2  Inertia=[1.25755e-06,0,0;0,1.41119e-07,0;0,0,1.16215e-06]  Shape=Cylinder  ShapeDims=[1 1]  ShapeUnits=m  ShapeUse=false  Density=1  DensityUnits=kg/m^3  DensityUse=false  GraphicsMode=GFXFILE  GraphicsFileName=MICROBOT_1 - W07-9.STL  BodyColorSelMode=COLORPALETTE  BodyColor=[0.792157;0.819608;0.933333]  AttachedToCS=CS1  CG=Right$CG$[-0.0592413 0.241684 0.239191]$WORLD$WORLD$m$[-0.430122 -0.898418 -0.0885398;-0.901961 0.431818 -3.2161e-12;0.0382331 0.0798594 -0.996073]$3x3 Transform$rad$WORLD$false$W07-9::CG(AUTOGEN)  WorkingFrames=Right$CS1$[-0.0587101 0.241684 0.245168]$WORLD$WORLD$m$[-0.430122 -0.898418 -0.0885398;-0.901961 0.431818 -3.2161e-12;0.0382331 0.0798594 -0.996073]$3x3 Transform$rad$WORLD$false$W07-9::CS1(AUTOGEN)#Left$CS2$[-0.0797149 0.251184 0.23298]$WORLD$WORLD$m$[1 0 0;0 1 0;0 0 1]$3x3 Transform$rad$WORLD$true$W06-4:-:W07-9::W07-9(AUTOGEN)#Right$CS3$[-0.0401844 0.232184 0.229466]$WORLD$WORLD$m$[1 0 0;0 1 0;0 0 1]$3x3 Transform$rad$WORLD$true$W07-9:-:W08-5::W07-9(AUTOGEN)  CGPos=[-0.0592413 0.241684 0.239191]  CGRot=[-0.430122 -0.898418 -0.0885398;-0.901961 0.431818 -3.2161e-12;0.0382331 0.0798594 -0.996073]  CS0Pos=[]  CS0Rot=[]  CS1Pos=[-0.0587101 0.241684 0.245168]  CS1Rot=[-0.430122 -0.898418 -0.0885398;-0.901961 0.431818 -3.2161e-12;0.0382331 0.0798594 -0.996073]  CS2Pos=[-0.0797149 0.251184 0.23298]  CS2Rot=[1 0 0;0 1 0;0 0 1]  CS3Pos=[-0.0401844 0.232184 0.229466]  CS3Rot=[1 0 0;0 1 0;0 0 1]  CS4Pos=[]  CS4Rot=[]  CS5Pos=[]  CS5Rot=[]  CS6Pos=[]  CS6Rot=[]  CS7Pos=[]  CS7Rot=[]  CS8Pos=[]  CS8Rot=[]  CS9Pos=[]  CS9Rot=[]  CS10Pos=[]  CS10Rot=[]  CS11Pos=[]  CS11Rot=[]  CS12Pos=[]  CS12Rot=[]  CS13Pos=[]  CS13Rot=[]  CS14Pos=[]  CS14Rot=[]  CS15Pos=[]  CS15Rot=[]  CS16Pos=[]  CS16Rot=[]  CS17Pos=[]  CS17Rot=[]  CS18Pos=[]  CS18Rot=[]  CS19Pos=[]  CS19Rot=[]  CS20Pos=[]  CS20Rot=[]
  W08-5 : mblibv1/Bodies/Body  LConnTagsString=CS2|CS3  UpdateFromCAD=on  PMImportedID=W08-5  DialogClass=MechanicalBodyBlock  Mass=0.000736673  MassUnits=kg  InertiaUnits=kg*m^2  Inertia=[7.2718e-08,9.77805e-09,0;9.77805e-09,5.45667e-08,0;0,0,4.04479e-08]  Shape=Cylinder  ShapeDims=[1 1]  ShapeUnits=m  ShapeUse=false  Density=1  DensityUnits=kg/m^3  DensityUse=false  GraphicsMode=GFXFILE  GraphicsFileName=MICROBOT_1 - W08-5.STL  BodyColorSelMode=COLORPALETTE  BodyColor=[0.792157;0.819608;0.933333]  AttachedToCS=CS1  CG=Right$CG$[-0.0309138 0.224849 0.237175]$WORLD$WORLD$m$[-1.35152e-12 -0.996073 -0.0885398;-1 1.64275e-12 -3.2164e-12;3.34921e-12 0.0885398 -0.996073]$3x3 Transform$rad$WORLD$false$W08-5::CG(AUTOGEN)  WorkingFrames=Right$CS1$[-0.0424201 0.221184 0.238198]$WORLD$WORLD$m$[-1.35152e-12 -0.996073 -0.0885398;-1 1.64275e-12 -3.2164e-12;3.34921e-12 0.0885398 -0.996073]$3x3 Transform$rad$WORLD$false$W08-5::CS1(AUTOGEN)#Left$CS2$[-0.0401844 0.232184 0.229466]$WORLD$WORLD$m$[1 0 0;0 1 0;0 0 1]$3x3 Transform$rad$WORLD$true$W07-9:-:W08-5::W08-5(AUTOGEN)#Left$CS3$[-0.0401844 0.224184 0.229466]$WORLD$WORLD$m$[1 0 0;0 1 0;0 0 1]$3x3 Transform$rad$WORLD$true$W07-10:-:W08-5::W08-5(AUTOGEN)  CGPos=[-0.0309138 0.224849 0.237175]  CGRot=[-1.35152e-12 -0.996073 -0.0885398;-1 1.64275e-12 -3.2164e-12;3.34921e-12 0.0885398 -0.996073]  CS0Pos=[]  CS0Rot=[]  CS1Pos=[-0.0424201 0.221184 0.238198]  CS1Rot=[-1.35152e-12 -0.996073 -0.0885398;-1 1.64275e-12 -3.2164e-12;3.34921e-12 0.0885398 -0.996073]  CS2Pos=[-0.0401844 0.232184 0.229466]  CS2Rot=[1 0 0;0 1 0;0 0 1]  CS3Pos=[-0.0401844 0.224184 0.229466]  CS3Rot=[1 0 0;0 1 0;0 0 1]  CS4Pos=[]  CS4Rot=[]  CS5Pos=[]  CS5Rot=[]  CS6Pos=[]  CS6Rot=[]  CS7Pos=[]  CS7Rot=[]  CS8Pos=[]  CS8Rot=[]  CS9Pos=[]  CS9Rot=[]  CS10Pos=[]  CS10Rot=[]  CS11Pos=[]  CS11Rot=[]  CS12Pos=[]  CS12Rot=[]  CS13Pos=[]  CS13Rot=[]  CS14Pos=[]  CS14Rot=[]  CS15Pos=[]  CS15Rot=[]  CS16Pos=[]  CS16Rot=[]  CS17Pos=[]  CS17Rot=[]  CS18Pos=[]  CS18Rot=[]  CS19Pos=[]  CS19Rot=[]  CS20Pos=[]  CS20Rot=[]
  W08-6 : mblibv1/Bodies/Body  LConnTagsString=CS2|CS3  UpdateFromCAD=on  PMImportedID=W08-6  DialogClass=MechanicalBodyBlock  Mass=0.000736673  MassUnits=kg  InertiaUnits=kg*m^2  Inertia=[7.2718e-08,9.77805e-09,0;9.77805e-09,5.45667e-08,0;0,0,4.04479e-08]  Shape=Cylinder  ShapeDims=[1 1]  ShapeUnits=m  ShapeUse=false  Density=1  DensityUnits=kg/m^3  DensityUse=false  GraphicsMode=GFXFILE  GraphicsFileName=MICROBOT_1 - W08-6.STL  BodyColorSelMode=COLORPALETTE  BodyColor=[0.792157;0.819608;0.933333]  AttachedToCS=CS1  CG=Right$CG$[-0.0309138 0.217519 0.237175]$WORLD$WORLD$m$[1.34788e-12 -0.996073 0.0885398;1 1.63919e-12 3.21743e-12;-3.34993e-12 0.0885398 0.996073]$3x3 Transform$rad$WORLD$false$W08-6::CG(AUTOGEN)  WorkingFrames=Right$CS1$[-0.0424201 0.221184 0.238198]$WORLD$WORLD$m$[1.34788e-12 -0.996073 0.0885398;1 1.63919e-12 3.21743e-12;-3.34993e-12 0.0885398 0.996073]$3x3 Transform$rad$WORLD$false$W08-6::CS1(AUTOGEN)#Left$CS2$[-0.0401844 0.218184 0.229466]$WORLD$WORLD$m$[1 0 0;0 1 0;0 0 1]$3x3 Transform$rad$WORLD$true$W07-11:-:W08-6::W08-6(AUTOGEN)#Left$CS3$[-0.0401844 0.210184 0.229466]$WORLD$WORLD$m$[1 0 0;0 1 0;0 0 1]$3x3 Transform$rad$WORLD$true$W07-12:-:W08-6::W08-6(AUTOGEN)  CGPos=[-0.0309138 0.217519 0.237175]  CGRot=[1.34788e-12 -0.996073 0.0885398;1 1.63919e-12 3.21743e-12;-3.34993e-12 0.0885398 0.996073]  CS0Pos=[]  CS0Rot=[]  CS1Pos=[-0.0424201 0.221184 0.238198]  CS1Rot=[1.34788e-12 -0.996073 0.0885398;1 1.63919e-12 3.21743e-12;-3.34993e-12 0.0885398 0.996073]  CS2Pos=[-0.0401844 0.218184 0.229466]  CS2Rot=[1 0 0;0 1 0;0 0 1]  CS3Pos=[-0.0401844 0.210184 0.229466]  CS3Rot=[1 0 0;0 1 0;0 0 1]  CS4Pos=[]  CS4Rot=[]  CS5Pos=[]  CS5Rot=[]  CS6Pos=[]  CS6Rot=[]  CS7Pos=[]  CS7Rot=[]  CS8Pos=[]  CS8Rot=[]  CS9Pos=[]  CS9Rot=[]  CS10Pos=[]  CS10Rot=[]  CS11Pos=[]  CS11Rot=[]  CS12Pos=[]  CS12Rot=[]  CS13Pos=[]  CS13Rot=[]  CS14Pos=[]  CS14Rot=[]  CS15Pos=[]  CS15Rot=[]  CS16Pos=[]  CS16Rot=[]  CS17Pos=[]  CS17Rot=[]  CS18Pos=[]  CS18Rot=[]  CS19Pos=[]  CS19Rot=[]  CS20Pos=[]  CS20Rot=[]
  Weld : mblibv1/Joints/Weld  LConnTagsString=__newl0  RConnTagsString=__newr0  UpdateFromCAD=on  PMImportedID=MICROBOT_1/RootPart:-:W03_1-1  NumSAPorts=0  CutJoint=off  MarkAsCut=off  Primitives=weld  PrimitiveProps=W$WORLD$[0.57735,0.57735,0.57735]$weld  DialogClass=JointBlock  WAxis=[0.57735,0.57735,0.57735]
  Weld1 : mblibv1/Joints/Weld  LConnTagsString=__newl0  RConnTagsString=__newr0  UpdateFromCAD=on  PMImportedID=W03_1-1:-:board-1  NumSAPorts=0  CutJoint=off  MarkAsCut=off  Primitives=weld  PrimitiveProps=W$WORLD$[0.57735,0.57735,0.57735]$weld  DialogClass=JointBlock  WAxis=[0.57735,0.57735,0.57735]
  Weld2 : mblibv1/Joints/Weld  LConnTagsString=__newl0  RConnTagsString=__newr0  UpdateFromCAD=on  PMImportedID=MICROBOT_1/RootPart:-:RootGround  NumSAPorts=0  CutJoint=off  MarkAsCut=off  Primitives=weld  PrimitiveProps=W$WORLD$[0.57735,0.57735,0.57735]$weld  DialogClass=JointBlock  WAxis=[0.57735,0.57735,0.57735]
  board-1 : mblibv1/Bodies/Body  LConnTagsString=CS2  UpdateFromCAD=on  PMImportedID=board-1  DialogClass=MechanicalBodyBlock  Mass=16.6499  MassUnits=kg  InertiaUnits=kg*m^2  Inertia=[0.354681,0.000443934,-0.000371852;0.000443934,0.564949,0.0503728;-0.000371852,0.0503728,0.428805]  Shape=Cylinder  ShapeDims=[1 1]  ShapeUnits=m  ShapeUse=false  Density=1  DensityUnits=kg/m^3  DensityUse=false  GraphicsMode=GFXFILE  GraphicsFileName=MICROBOT_1 - board-1.STL  BodyColorSelMode=COLORPALETTE  BodyColor=[0.792157;0.819608;0.933333]  AttachedToCS=CS1  CG=Right$CG$[-0.103889 0.511188 0.036415]$WORLD$WORLD$m$[1 0 0;0 0 -1;0 1 0]$3x3 Transform$rad$WORLD$false$board-1::CG(AUTOGEN)  WorkingFrames=Right$CS1$[-0.103779 0.498684 -0.02]$WORLD$WORLD$m$[1 0 0;0 0 -1;0 1 0]$3x3 Transform$rad$WORLD$false$board-1::CS1(AUTOGEN)#Left$CS2$[-0.107087 0.036184 -0.02]$WORLD$WORLD$m$[1 0 0;0 1 0;0 0 1]$3x3 Transform$rad$WORLD$true$W03_1-1:-:board-1::board-1(AUTOGEN)  CGPos=[-0.103889 0.511188 0.036415]  CGRot=[1 0 0;0 0 -1;0 1 0]  CS0Pos=[]  CS0Rot=[]  CS1Pos=[-0.103779 0.498684 -0.02]  CS1Rot=[1 0 0;0 0 -1;0 1 0]  CS2Pos=[-0.107087 0.036184 -0.02]  CS2Rot=[1 0 0;0 1 0;0 0 1]  CS3Pos=[]  CS3Rot=[]  CS4Pos=[]  CS4Rot=[]  CS5Pos=[]  CS5Rot=[]  CS6Pos=[]  CS6Rot=[]  CS7Pos=[]  CS7Rot=[]  CS8Pos=[]  CS8Rot=[]  CS9Pos=[]  CS9Rot=[]  CS10Pos=[]  CS10Rot=[]  CS11Pos=[]  CS11Rot=[]  CS12Pos=[]  CS12Rot=[]  CS13Pos=[]  CS13Rot=[]  CS14Pos=[]  CS14Rot=[]  CS15Pos=[]  CS15Rot=[]  CS16Pos=[]  CS16Rot=[]  CS17Pos=[]  CS17Rot=[]  CS18Pos=[]  CS18Rot=[]  CS19Pos=[]  CS19Rot=[]  CS20Pos=[]  CS20Rot=[]
  wires:
  Constant/1 -> Mux/1
  Constant21/1 -> Subsystem5/3(id)
  Constant6/1 -> Subsystem5/2(delay)
  Subsystem5/1(Out1) -> Display6/1
  Constant25/1 -> Subsystem5/1(k)
  Constant20/1 -> Mux6/3
  Constant19/1 -> Mux6/2
  Mux6/1 -> Joint Actuator1/1
  Constant1/1 -> Mux6/1
  Constant18/1 -> Mux5/3
  Constant17/1 -> Mux5/2
  Mux5/1 -> Joint Actuator6/1
  Constant22/1 -> Mux5/1
  Constant16/1 -> Mux4/3
  Constant15/1 -> Mux4/2
  Mux4/1 -> Joint Actuator5/1
  Constant5/1 -> Mux4/1
  Constant14/1 -> Mux3/3
  Constant13/1 -> Mux3/2
  Mux3/1 -> Joint Actuator4/1
  Constant4/1 -> Mux3/1
  Constant12/1 -> Mux2/3
  Constant11/1 -> Mux2/2
  Mux2/1 -> Joint Actuator3/1
  Constant3/1 -> Mux2/1
  Constant10/1 -> Mux1/3
  Constant9/1 -> Mux1/2
  Mux1/1 -> Joint Actuator2/1
  Constant2/1 -> Mux1/1
  Constant8/1 -> Mux/3
  Constant7/1 -> Mux/2
  Mux/1 -> Joint Actuator/1
  connections:
  Revolute7/LConn2 -- Joint Actuator1/RConn1
  Joint Actuator6/RConn1 -- Revolute5/LConn2
  Joint Actuator5/RConn1 -- Revolute1/LConn2
  Joint Actuator4/RConn1 -- Revolute/LConn2
  Joint Actuator3/RConn1 -- Revolute3/LConn2
  Revolute8/LConn2 -- Joint Actuator2/RConn1
  Joint Actuator/RConn1 -- Revolute4/LConn2
  RootGround/LConn1 -- Machine Environment/RConn1
  RootPart/RConn1 -- Weld/LConn1
  Weld/RConn1 -- W03_1-1/LConn1
  W07-11/RConn1 -- Cylindrical1/LConn1
  Cylindrical1/RConn1 -- W08-6/LConn1
  W06-4/RConn1 -- Revolute5/LConn1
  Revolute5/RConn1 -- W07-11/LConn1
  W01_2-2/RConn1 -- Revolute8/LConn1
  Revolute8/RConn1 -- W02_1-3/LConn1
  W03_1-1/RConn1 -- Revolute4/LConn1
  Revolute4/RConn1 -- W01_2-2/LConn1
  W02_1-3/RConn1 -- Revolute3/LConn1
  Revolute3/RConn1 -- W04-3/LConn1
  W07-12/RConn1 -- Revolute10/LConn1
  Revolute10/RConn1 -- W08-6/LConn2
  W04-3/RConn1 -- Revolute/LConn1
  Revolute/RConn1 -- W05-4/LConn1
  W05-4/RConn1 -- Revolute1/LConn1
  Revolute1/RConn1 -- W06-4/LConn1
  W06-4/RConn2 -- Revolute6/LConn1
  Revolute6/RConn1 -- W07-12/LConn1
  W06-4/RConn3 -- Revolute2/LConn1
  Revolute2/RConn1 -- W07-9/LConn1
  W06-4/RConn4 -- Revolute7/LConn1
  Revolute7/RConn1 -- W07-10/LConn1
  W03_1-1/RConn2 -- Weld1/LConn1
  Weld1/RConn1 -- board-1/LConn1
  W07-9/RConn1 -- Cylindrical/LConn1
  Cylindrical/RConn1 -- W08-5/LConn1
  W07-10/RConn1 -- Revolute9/LConn1
  Revolute9/RConn1 -- W08-5/LConn2
  RootGround/RConn1 -- Weld2/LConn1
  Weld2/RConn1 -- RootPart/LConn1

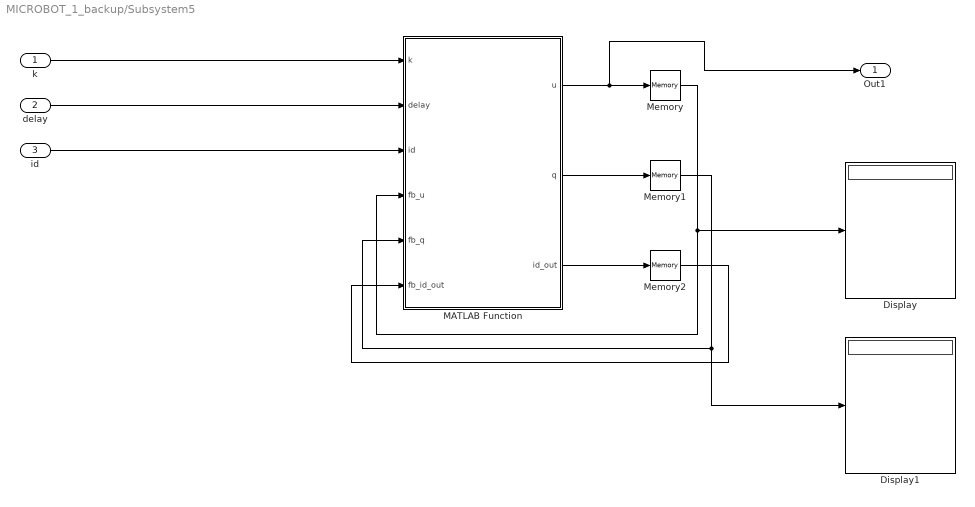
== system MICROBOT_1_backup/Subsystem5 ==
  k : Inport
  delay : Inport  Port=2
  id : Inport  Port=3
  Display : Display
  Display1 : Display
  MATLAB Function : MATLAB Function  TreatAsAtomicUnit=on
  Memory : Memory  X0=[0, 0 ,0, 0, 0, 0]
  Memory1 : Memory  X0=[0, 0 ,0, 0, 0, 0]
  Memory2 : Memory
  Out1 : Outport
  wires:
  k/1 -> MATLAB Function/1(k)
  delay/1 -> MATLAB Function/2(delay)
  MATLAB Function/1(u) -> Out1/1, Memory/1
  MATLAB Function/2(q) -> Memory1/1
  MATLAB Function/3(id_out) -> Memory2/1
  Memory/1 -> Display/1, MATLAB Function/4(fb_u)
  Memory1/1 -> Display1/1, MATLAB Function/5(fb_q)
  id/1 -> MATLAB Function/3(id)
  Memory2/1 -> MATLAB Function/6(fb_id_out)

== matlab function MICROBOT_1_backup/Subsystem5/MATLAB Function ==
  data: u output; k input; q output; delay input; id input; fb_u input; fb_q input; id_out output; fb_id_out input
function [u, q, id_out] = fcn(k, delay, id, fb_u, fb_q, fb_id_out)
%#codegen  
    
    temp1 = fb_u;
    temp2 = fb_q;
    ts = 0.03;
    ns = delay / ts;
    if fb_id_out == id
        for i = 1:6
            if fb_q(i) < abs(k(i))
                temp1(i) = fb_u(i) + k(i) / ns;
                temp2(i) = fb_q(i) + abs(k(i) / ns);              
            else
                temp1(i) = fb_u(i);
            end
        end
    else
        for i = 1:6
            temp2(i) = 0;
        end
    end

% pause(ts*0.05);
u = temp1;
q = temp2;
id_out = id;
